simulink model "storage_test"  (R2023b)
settings: Solver=ode15s  StartTime=0.0  StopTime=200  FixedStep=0.01  RelTol=1e-5  AbsTol=1e-8
values from neighbouring files (symbols this model uses):
  ACTIVATE = [ 0 ]    [init_bsm1.m]    (also in init_bsm2.m)
  Qstorage = 0    [reginit_bsm1.m]    (also in reginit_bsm2.m)
  TEMPMODEL = [ 0 ]    [init_bsm1.m]    (also in init_bsm2.m)
undefined symbols (not defined in the file or in its folder): TIMEDELAY_S, VOL_INIT_S, VOL_S, XINITSTORAGE
settings Model: Creator=ielulf  LastModifiedBy=BuB
settings SolverCC: AutoScaleAbsTol=off  AlgebraicLoopSolver=TrustRegion
settings DataIOCC: InitialState=xFinal  SaveFormat=Array  SignalLoggingSaveFormat=ModelDataLogs  SaveOutput=off  ReturnWorkspaceOutputs=off  TimeSaveName=t  SignalLoggingName=sigsOut  OutputTimes=[0:(1/96):609]
settings OptimizationCC: BlockReduction=off  BooleanDataType=off  OptimizeBlockIOStorage=off  BufferReuse=off  GlobalBufferReuse=off  ExpressionFolding=off  LocalBlockOutputs=off  InitFltsAndDblsToZero=on  LifeSpan=inf  OptimizeDataStoreBuffers=off  BusAssignmentInplaceUpdate=off
settings DebuggingCC: SaveWithParameterizedLinksMsg=none  UnderspecifiedInitializationDetection=Classic  MergeDetectMultiDrivingBlocksExec=none  SignalResolutionControl=TryResolveAllWithWarning  InheritedTsInSrcMsg=none  MultiTaskDSMMsg=warning  MultiTaskCondExecSysMsg=none  FcnCallInpInsideContextMsg=warning  UnconnectedInputMsg=warning  UnconnectedLineMsg=warning  SFUnexpectedBacktrackingDiag=warning  SFNoUnconditionalDefaultTransitionDiag=warning  SFExecutionAtInitializationDiag=none  ArithmeticOperatorsInVariantConditions=warning
settings HardwareCC: ProdBitPerPointer=32  ProdBitPerSizeT=32  ProdBitPerPtrDiffT=32  ProdLargestAtomicFloat=None  ProdIntDivRoundTo=Undefined  ProdEndianess=Unspecified  ProdWordSize=32  ProdHWDeviceType=32-bit Generic  TargetUnknown=on
settings ModelReferenceCC: EnableRefExpFcnMdlSchedulingChecks=on  PropagateSignalLabelsOutOfModel=off
settings RTWCC: TemplateMakefile=grt_unix.tmf
settings CodeAppCC: StateflowObjectComments=on
settings GRTTargetCC: TargetFcnLib=ansi_tfl_tmw.mat  TargetLangStandard=C89/C90 (ANSI)  CombineOutputUpdateFcns=off  GRTInterface=on
settings ConfigComp: CovMetricSettings=dw  CovSaveCumulativeToWorkspaceVar=on  CovSaveSingleToWorkspaceVar=on

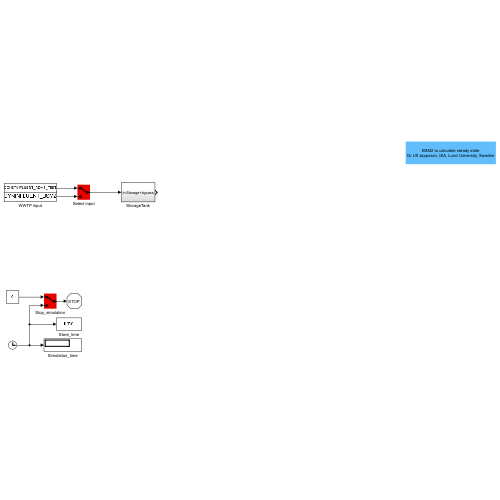
[thumbnail: Simulink's stored preview of the top-level diagram]
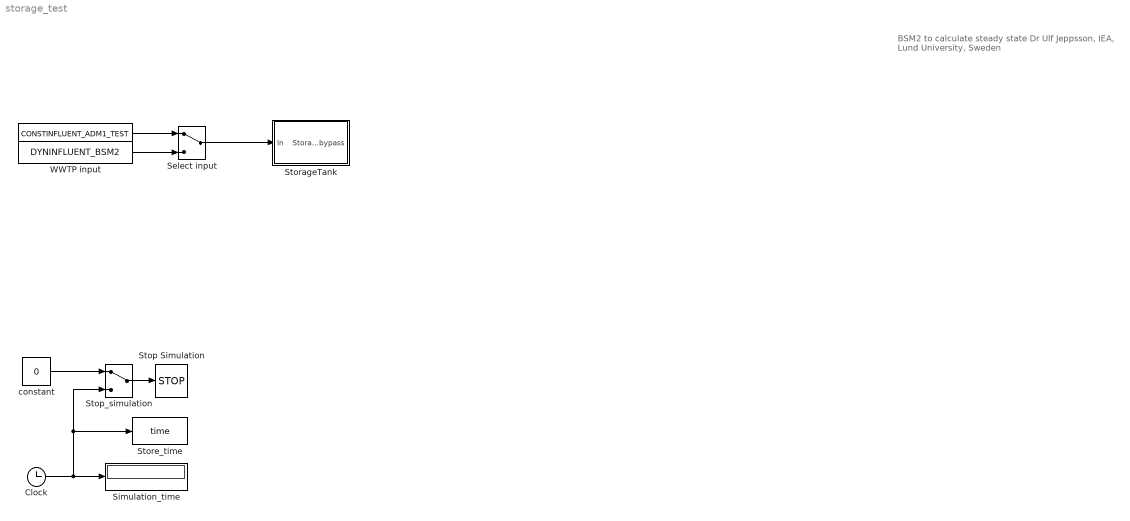
== system storage_test ==
  note: BSM2 to calculate steady state
      |  Dr Ulf Jeppsson, IEA, Lund University, Sweden
  " " : FromWorkspace  VariableName=CONSTINFLUENT_ADM1_TEST  SampleTime=-1  ZeroCross=off  OutputAfterFinalValue=Holding final value
  " constant" : Constant  Value=0
  Clock : Clock
  Select input : ManualSwitch
  Simulation_time : Display
  Stop Simulation : Stop
  Stop_simulation : ManualSwitch
  StorageTank : Subsystem
  Store_time : ToWorkspace  VariableName=time
  WWTP input : FromWorkspace  VariableName=DYNINFLUENT_BSM2  SampleTime=-1  ZeroCross=off  OutputAfterFinalValue=Holding final value
  wires:
  Clock/1 -> Simulation_time/1, Stop_simulation/2, Store_time/1
  Stop_simulation/1 -> Stop Simulation/1
  " constant"/1 -> Stop_simulation/1
  Select input/1 -> StorageTank/1(In)
  " "/1 -> Select input/1
  WWTP input/1 -> Select input/2

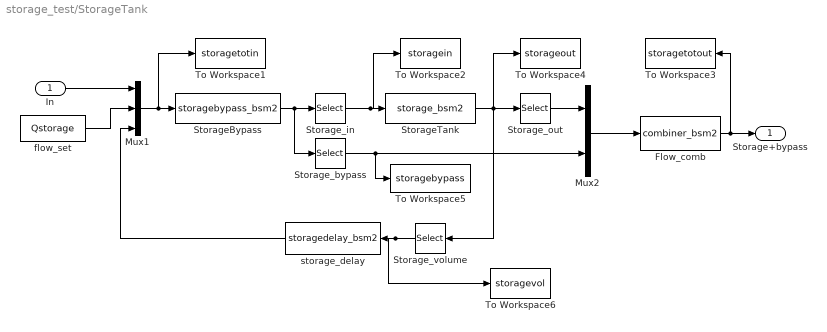
== system storage_test/StorageTank ==
  In : Inport
  Flow_comb : S-Function  FunctionName=combiner_bsm2  SFunctionDeploymentMode=off  EnableBusSupport=off
  Mux1 : Mux  Inputs=3
  Mux2 : Mux  Inputs=2
  StorageBypass : S-Function  FunctionName=storagebypass_bsm2  Parameters=VOL_S  SFunctionDeploymentMode=off  EnableBusSupport=off
  StorageTank : S-Function  FunctionName=storage_bsm2  Parameters=XINITSTORAGE,VOL_S,TEMPMODEL,ACTIVATE  SFunctionDeploymentMode=off  EnableBusSupport=off
  Storage_bypass : Selector  InputPortWidth=43  IndexOptions=Index vector (dialog)  Indices=[23:43]  OutputSizes=1
  Storage_in : Selector  InputPortWidth=43  IndexOptions=Index vector (dialog)  Indices=[1:22]  OutputSizes=1
  Storage_out : Selector  InputPortWidth=22  IndexOptions=Index vector (dialog)  Indices=[1:21]  OutputSizes=1
  Storage_volume : Selector  InputPortWidth=22  IndexOptions=Index vector (dialog)  Indices=[22]  OutputSizes=1
  To Workspace1 : ToWorkspace  VariableName=storagetotin
  To Workspace2 : ToWorkspace  VariableName=storagein
  To Workspace3 : ToWorkspace  VariableName=storagetotout
  To Workspace4 : ToWorkspace  VariableName=storageout
  To Workspace5 : ToWorkspace  VariableName=storagebypass
  To Workspace6 : ToWorkspace  VariableName=storagevol
  flow_set : Constant  Value=Qstorage
  storage_delay : S-Function  FunctionName=storagedelay_bsm2  Parameters=VOL_INIT_S,TIMEDELAY_S  SFunctionDeploymentMode=off  EnableBusSupport=off
  Storage+bypass : Outport
  wires:
  Flow_comb/1 -> Storage+bypass/1, To Workspace3/1
  Storage_volume/1 -> To Workspace6/1, storage_delay/1
  In/1 -> Mux1/1
  Storage_out/1 -> Mux2/1
  StorageTank/1 -> Storage_volume/1, To Workspace4/1, Storage_out/1
  Storage_bypass/1 -> To Workspace5/1, Mux2/2
  Storage_in/1 -> To Workspace2/1, StorageTank/1
  Mux2/1 -> Flow_comb/1
  StorageBypass/1 -> Storage_bypass/1, Storage_in/1
  flow_set/1 -> Mux1/2
  Mux1/1 -> To Workspace1/1, StorageBypass/1
  storage_delay/1 -> Mux1/3
